simulink model "ESTS_test"  (R2024b)
settings: Solver=VariableStepAuto  StartTime=0.0  StopTime=10.0  RelTol=1e-3
libraries: ESTS x1
settings Model: Creator=blatak  LastModifiedBy=blatak

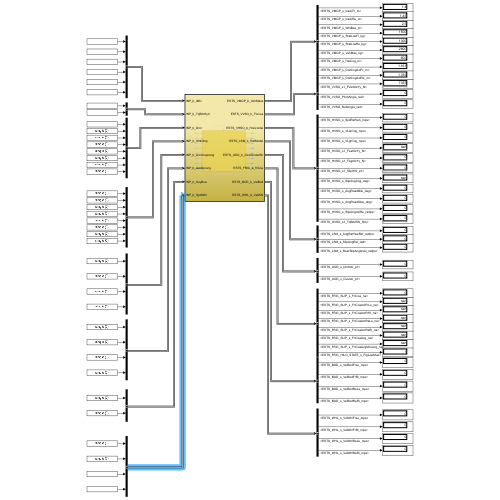
[thumbnail: Simulink's stored preview of the top-level diagram]
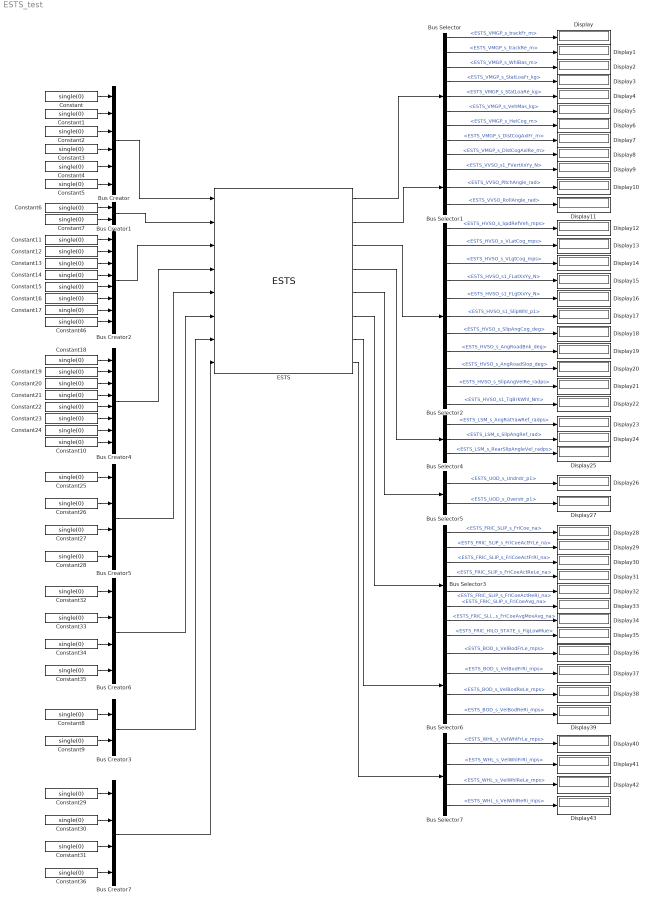
== system ESTS_test ==
  Bus Creator : BusCreator  Inputs=6  OutDataTypeStr=Bus: INP_b_IMU
      settings: InheritFromInputs=off
  Bus Creator1 : BusCreator  Inputs=2  OutDataTypeStr=Bus: INP_b_TqBrkHyd
      settings: InheritFromInputs=off
  Bus Creator2 : BusCreator  Inputs=8  OutDataTypeStr=Bus: INP_b_Drvr
      settings: InheritFromInputs=off
  Bus Creator3 : BusCreator  Inputs=2  OutDataTypeStr=Bus: INP_b_KeyBoa
      settings: InheritFromInputs=off
  Bus Creator4 : BusCreator  Inputs=8  OutDataTypeStr=Bus: INP_b_StrkDmp
      settings: InheritFromInputs=off
  Bus Creator5 : BusCreator  Inputs=4  OutDataTypeStr=Bus: INP_b_AccUnsp
      settings: InheritFromInputs=off
  Bus Creator6 : BusCreator  Inputs=4  OutDataTypeStr=Bus: INP_b_AccSpr
      settings: InheritFromInputs=off
  Bus Creator7 : BusCreator  Inputs=4  OutDataTypeStr=Bus: INP_b_SpdWhl
      settings: InheritFromInputs=off
  Bus Selector : BusSelector  OutputSignals=ESTS_VMGP_s_trackFr_m,ESTS_VMGP_s_trackRe_m,ESTS_VMGP_s_WhlBas_m,ESTS_VMGP_s_StatLoaFr_kg,ESTS_VMGP_s_StatLoaRe_kg,ESTS_VMGP_s_VehMas_kg,ESTS_VMGP_s_HeiCog_m,ESTS_VMGP_s_DistCogAxlFr_m,ESTS_VMGP_s_DistCogAxlRe_m
  Bus Selector1 : BusSelector  OutputSignals=ESTS_VVSO_s1_FVertXxYy_N,ESTS_VVSO_PitchAngle_rad,ESTS_VVSO_RollAngle_rad
  Bus Selector2 : BusSelector  OutputSignals=ESTS_HVSO_s_SpdRefVeh_mps,ESTS_HVSO_s_VLatCog_mps,ESTS_HVSO_s_VLgtCog_mps,ESTS_HVSO_s1_FLatXxYy_N,ESTS_HVSO_s1_FLgtXxYy_N,ESTS_HVSO_s1_SlipWhl_p1,ESTS_HVSO_s_SlipAngCog_deg,ESTS_HVSO_s_AngRoadBnk_deg,ESTS_HVSO_s_AngRoadSlop_deg,ESTS_HVSO_s_SlipAngVelRe_radps,ESTS_HVSO_s1_TqBrkWhl_Nm
  Bus Selector3 : BusSelector  OutputSignals=ESTS_FRIC_SLIP_s_FriCoe_na,ESTS_FRIC_SLIP_s_FriCoeActFrLe_na,ESTS_FRIC_SLIP_s_FriCoeActFrRi_na,ESTS_FRIC_SLIP_s_FriCoeActReLe_na,ESTS_FRIC_SLIP_s_FriCoeActReRi_na,ESTS_FRIC_SLIP_s_FriCoeAvg_na,ESTS_FRIC_SLIP_s_FriCoeAvgMovAvg_na,ESTS_FRIC_HILO_STATE_s_FlgLowMue
  Bus Selector4 : BusSelector  OutputSignals=ESTS_LSM_s_AngRatYawRef_radps,ESTS_LSM_s_SlipAngRef_rad,ESTS_LSM_s_RearSlipAngleVel_radps
  Bus Selector5 : BusSelector  OutputSignals=ESTS_UOD_s_Undrstr_p1,ESTS_UOD_s_Overstr_p1
  Bus Selector6 : BusSelector  OutputSignals=ESTS_BOD_s_VelBodFrLe_mps,ESTS_BOD_s_VelBodFrRi_mps,ESTS_BOD_s_VelBodReLe_mps,ESTS_BOD_s_VelBodReRi_mps
  Bus Selector7 : BusSelector  OutputSignals=ESTS_WHL_s_VelWhlFrLe_mps,ESTS_WHL_s_VelWhlFrRi_mps,ESTS_WHL_s_VelWhlReLe_mps,ESTS_WHL_s_VelWhlReRi_mps
  Constant{,1..36,46} (38 alike) : Constant  Value=single(0)
  Display{,1..43} (44 alike) : Display
  ESTS : ESTS/ESTS  SystemSampleTime=-1  VariantActivationTime=update diagram  AllowFlexibleInterface=on  Latency=0  AutoFrameSizeCalculation=off
  wires:
  ESTS/6 -> Bus Selector3/1
  ESTS/1 -> Bus Selector/1
  ESTS/2 -> Bus Selector1/1
  ESTS/3 -> Bus Selector2/1
  ESTS/4 -> Bus Selector4/1
  ESTS/5 -> Bus Selector5/1
  Bus Selector/1 -> Display/1  "<ESTS_VMGP_s_trackFr_m>"
  Bus Selector/2 -> Display1/1  "<ESTS_VMGP_s_trackRe_m>"
  Bus Selector/3 -> Display2/1  "<ESTS_VMGP_s_WhlBas_m>"
  Bus Selector/4 -> Display3/1  "<ESTS_VMGP_s_StatLoaFr_kg>"
  Bus Selector/5 -> Display4/1  "<ESTS_VMGP_s_StatLoaRe_kg>"
  Bus Selector/6 -> Display5/1  "<ESTS_VMGP_s_VehMas_kg>"
  Bus Selector/7 -> Display6/1  "<ESTS_VMGP_s_HeiCog_m>"
  Bus Selector/9 -> Display8/1  "<ESTS_VMGP_s_DistCogAxlRe_m>"
  Bus Selector/8 -> Display7/1  "<ESTS_VMGP_s_DistCogAxlFr_m>"
  Bus Selector1/1 -> Display9/1  "<ESTS_VVSO_s1_FVertXxYy_N>"
  Bus Selector1/2 -> Display10/1  "<ESTS_VVSO_PitchAngle_rad>"
  Bus Selector1/3 -> Display11/1  "<ESTS_VVSO_RollAngle_rad>"
  Bus Selector2/1 -> Display12/1  "<ESTS_HVSO_s_SpdRefVeh_mps>"
  Bus Selector2/10 -> Display21/1  "<ESTS_HVSO_s_SlipAngVelRe_radps>"
  Bus Selector2/2 -> Display13/1  "<ESTS_HVSO_s_VLatCog_mps>"
  Bus Selector2/3 -> Display14/1  "<ESTS_HVSO_s_VLgtCog_mps>"
  Bus Selector2/4 -> Display15/1  "<ESTS_HVSO_s1_FLatXxYy_N>"
  Bus Selector2/5 -> Display16/1  "<ESTS_HVSO_s1_FLgtXxYy_N>"
  Bus Selector2/6 -> Display17/1  "<ESTS_HVSO_s1_SlipWhl_p1>"
  Bus Selector2/7 -> Display18/1  "<ESTS_HVSO_s_SlipAngCog_deg>"
  Bus Selector2/8 -> Display19/1  "<ESTS_HVSO_s_AngRoadBnk_deg>"
  Bus Selector2/9 -> Display20/1  "<ESTS_HVSO_s_AngRoadSlop_deg>"
  Bus Selector2/11 -> Display22/1  "<ESTS_HVSO_s1_TqBrkWhl_Nm>"
  Bus Selector4/1 -> Display23/1  "<ESTS_LSM_s_AngRatYawRef_radps>"
  Bus Selector4/2 -> Display24/1  "<ESTS_LSM_s_SlipAngRef_rad>"
  Bus Selector4/3 -> Display25/1  "<ESTS_LSM_s_RearSlipAngleVel_radps>"
  Bus Selector5/2 -> Display27/1  "<ESTS_UOD_s_Overstr_p1>"
  Bus Selector5/1 -> Display26/1  "<ESTS_UOD_s_Undrstr_p1>"
  Bus Selector3/1 -> Display28/1  "<ESTS_FRIC_SLIP_s_FriCoe_na>"
  Bus Selector3/2 -> Display29/1  "<ESTS_FRIC_SLIP_s_FriCoeActFrLe_na>"
  Bus Selector3/7 -> Display34/1  "<ESTS_FRIC_SLIP_s_FriCoeAvgMovAvg_na>"
  Bus Selector3/8 -> Display35/1  "<ESTS_FRIC_HILO_STATE_s_FlgLowMue>"
  Bus Selector3/6 -> Display33/1  "<ESTS_FRIC_SLIP_s_FriCoeAvg_na>"
  Bus Selector3/5 -> Display32/1  "<ESTS_FRIC_SLIP_s_FriCoeActReRi_na>"
  Bus Selector3/4 -> Display31/1  "<ESTS_FRIC_SLIP_s_FriCoeActReLe_na>"
  Bus Selector3/3 -> Display30/1  "<ESTS_FRIC_SLIP_s_FriCoeActFrRi_na>"
  Constant/1 -> Bus Creator/1
  Constant1/1 -> Bus Creator/2
  Constant2/1 -> Bus Creator/3
  Constant3/1 -> Bus Creator/4
  Constant4/1 -> Bus Creator/5
  Constant5/1 -> Bus Creator/6
  Constant6/1 -> Bus Creator1/1
  Constant7/1 -> Bus Creator1/2
  Constant8/1 -> Bus Creator3/1
  Constant9/1 -> Bus Creator3/2
  Constant11/1 -> Bus Creator2/1
  Constant12/1 -> Bus Creator2/2
  Constant13/1 -> Bus Creator2/3
  Constant14/1 -> Bus Creator2/4
  Constant16/1 -> Bus Creator2/6
  Constant17/1 -> Bus Creator2/7
  Constant18/1 -> Bus Creator4/1
  Constant19/1 -> Bus Creator4/2
  Constant25/1 -> Bus Creator5/1
  Constant26/1 -> Bus Creator5/2
  Constant27/1 -> Bus Creator5/3
  Constant32/1 -> Bus Creator6/1
  Constant33/1 -> Bus Creator6/2
  Constant34/1 -> Bus Creator6/3
  Constant35/1 -> Bus Creator6/4
  Bus Creator/1 -> ESTS/1
  Bus Creator1/1 -> ESTS/2
  Constant15/1 -> Bus Creator2/5
  Bus Creator4/1 -> ESTS/4
  Bus Creator5/1 -> ESTS/5
  Bus Creator6/1 -> ESTS/6
  Bus Creator3/1 -> ESTS/7
  Bus Selector6/1 -> Display36/1  "<ESTS_BOD_s_VelBodFrLe_mps>"
  ESTS/7 -> Bus Selector6/1
  ESTS/8 -> Bus Selector7/1
  Bus Selector7/1 -> Display40/1  "<ESTS_WHL_s_VelWhlFrLe_mps>"
  Bus Selector7/2 -> Display41/1  "<ESTS_WHL_s_VelWhlFrRi_mps>"
  Bus Selector7/3 -> Display42/1  "<ESTS_WHL_s_VelWhlReLe_mps>"
  Bus Selector7/4 -> Display43/1  "<ESTS_WHL_s_VelWhlReRi_mps>"
  Bus Selector6/2 -> Display37/1  "<ESTS_BOD_s_VelBodFrRi_mps>"
  Bus Selector6/3 -> Display38/1  "<ESTS_BOD_s_VelBodReLe_mps>"
  Bus Selector6/4 -> Display39/1  "<ESTS_BOD_s_VelBodReRi_mps>"
  Constant46/1 -> Bus Creator2/8
  Bus Creator2/1 -> ESTS/3
  Constant20/1 -> Bus Creator4/3
  Constant21/1 -> Bus Creator4/4
  Constant22/1 -> Bus Creator4/5
  Constant23/1 -> Bus Creator4/6
  Constant24/1 -> Bus Creator4/7
  Constant10/1 -> Bus Creator4/8
  Constant28/1 -> Bus Creator5/4
  Constant30/1 -> Bus Creator7/2
  Constant31/1 -> Bus Creator7/3
  Constant29/1 -> Bus Creator7/1
  Constant36/1 -> Bus Creator7/4
  Bus Creator7/1 -> ESTS/8
